simulink model "Team_46"  (R2021a)
settings: Solver=VariableStepAuto  StartTime=0.0  StopTime=1.79  RelTol=1e-3
undefined symbols (not defined in the file): D1, Delta
libraries: spsLoadFlowBusLib x5, spsThreePhaseVIMeasurementLib x4, spsThreePhaseSeriesRLCBranchLib x3, spsThreePhaseParallelRLCLoadLib x3, spsMultimeterLib x3, spsThreePhaseSourceLib x2, spsThreePhaseFaultLib x2, spsSynchronousMachinepuStandardLib x2, spsThreePhaseTransformerTwoWindingsLib x2, spsThreePhaseMutualInductanceZ1Z0Lib x2, spsThreePhaseSeriesRLCLoadLib x1, spsParallelRLCBranchLib x1
settings Model: Creator=Tanvi Purwar  LastModifiedBy=Tanvi Purwar

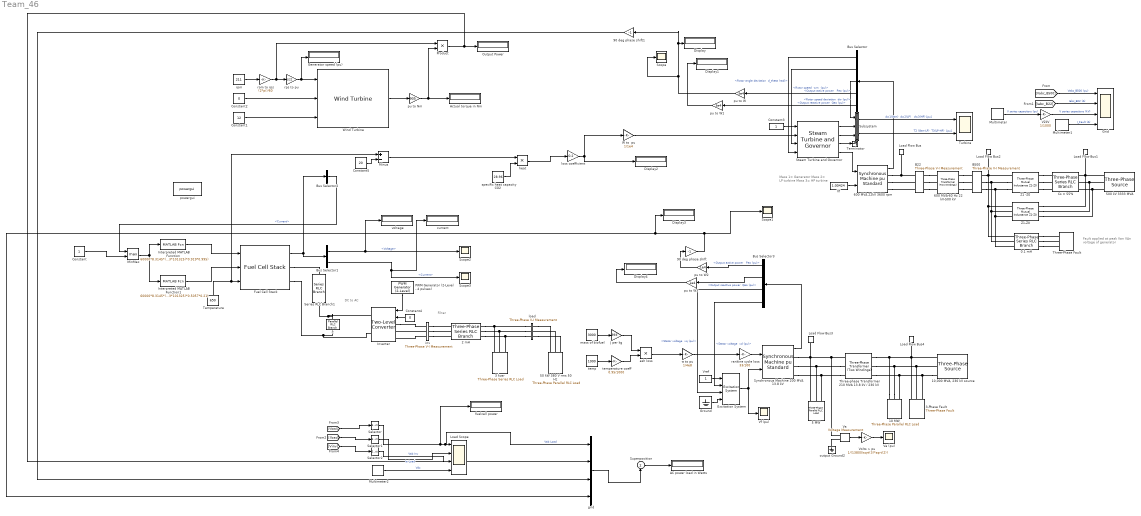
== system Team_46 ==
  note: DC to AC
  note: Mass 1= Generator
      | Mass 2= LP turbine
      | Mass 3= HP turbine
  note: Fault applied at peak Van
      | VAn voltage of generator
  note: Filter
  " mass of biofuel" : Constant  Value=3000
  0.1 mH : spsThreePhaseSeriesRLCBranchLib/Three-Phase Series RLC Branch  LConnTagsString=A|B|C  RConnTagsString=A|B|C  BranchType=L  Resistance=1.0  Inductance=0.1e-3  Capacitance=1e-6  Measurements=None
  10 MW : spsThreePhaseParallelRLCLoadLib/Three-Phase Parallel RLC Load  LConnTagsString=A|B|C  Configuration=Y (grounded)  NominalVoltage=230e3  Vabc=[1e3 1e3 1e3]  Vabcp=[1e3 1e3 1e3]  NominalFrequency=60  UnbalancedPower=off  ActivePower=10000000  InductivePower=0  CapacitivePower=0  Pabc=[10e3 9e3 11e3]  QLabc=[100 90 110]  QCabc=[100 90 110]  Pabcp=[10e3 9e3 11e3]  QLabcp=[100 90 110]  QCabcp=[100 90 110]  Measurements=None  LoadType=constant Z
  "10,000 MVA, 230 kV source" : spsThreePhaseSourceLib/Three-Phase Source  InternalConnection=Yg  VoltagePhases=off  Voltage=(230000)*1.00006  PhaseAngle=-0.77547  Voltage_phases=[25e3 25e3 25e3]/sqrt(3)  PhaseAngles_phases=[0 -120 +120]  Frequency=60  NonIdealSource=on  SpecifyImpedance=on  Resistance=0.529  Inductance=0.0140  ShortCircuitLevel=10000e6  BaseVoltage=230e3  XRratio=10  BusType=swing  Pref=0  Qref=0  Prefabc=[10e3, 10e3, 10e3]  Qrefabc=[0, 0, 0]  Qmin=-Inf  Qmax=Inf
  "2 mH " : spsThreePhaseSeriesRLCBranchLib/Three-Phase Series RLC Branch  LConnTagsString=A|B|C  RConnTagsString=A|B|C  BranchType=L  Resistance=0  Inductance=2e-3  Capacitance=inf  Measurements=None
  3 kvar : spsThreePhaseSeriesRLCLoadLib/Three-Phase Series RLC Load  LConnTagsString=A|B|C  Configuration=Delta  NominalVoltage=380  Vabc=[1e3 1e3 1e3]  Vabcp=[1e3 1e3 1e3]  NominalFrequency=50  UnbalancedPower=off  ActivePower=0  InductivePower=0  CapacitivePower=3e3  Pabc=[10e3 9e3 11e3]  QLabc=[100 90 110]  QCabc=[100 90 110]  Pabcp=[10e3 9e3 11e3]  QLabcp=[100 90 110]  QCabcp=[100 90 110]  Measurements=None  LoadType=constant Z
  3-Phase Fault : spsThreePhaseFaultLib/Three-Phase Fault  InitialStates=0  FaultA=on  FaultB=on  FaultC=on  GroundFault=on  SwitchTimes=[ 0.1 0.2]  External=off  SwitchStatus=NaN  FaultResistance=1e-3  GroundResistance=1e-3  SnubberResistance=inf  SnubberCapacitance=inf  Measurements=None
  5 MW : spsThreePhaseParallelRLCLoadLib/Three-Phase Parallel RLC Load  LConnTagsString=A|B|C  Configuration=Y (grounded)  NominalVoltage=13.8e3  Vabc=[1e3 1e3 1e3]  Vabcp=[1e3 1e3 1e3]  NominalFrequency=60  UnbalancedPower=off  ActivePower=5000000  InductivePower=0  CapacitivePower=0  Pabc=[10e3 9e3 11e3]  QLabc=[100 90 110]  QCabc=[100 90 110]  Pabcp=[10e3 9e3 11e3]  QLabcp=[100 90 110]  QCabcp=[100 90 110]  Measurements=None  LoadType=constant Z
  50 kW 380 V rms 50 Hz : spsThreePhaseParallelRLCLoadLib/Three-Phase Parallel RLC Load  LConnTagsString=A|B|C  Configuration=Delta  NominalVoltage=380  Vabc=[1e3 1e3 1e3]  Vabcp=[1e3 1e3 1e3]  NominalFrequency=50  UnbalancedPower=off  ActivePower=50e3  InductivePower=0  CapacitivePower=0  Pabc=[10e3 9e3 11e3]  QLabc=[100 90 110]  QCabc=[100 90 110]  Pabcp=[10e3 9e3 11e3]  QLabcp=[100 90 110]  QCabcp=[100 90 110]  Measurements=None  LoadType=constant Z
  500 kV 3333 MVA : spsThreePhaseSourceLib/Three-Phase Source  InternalConnection=Yg  VoltagePhases=off  Voltage=(500000)*0.99995  PhaseAngle=0.063884  Voltage_phases=[25e3 25e3 25e3]/sqrt(3)  PhaseAngles_phases=[0 -120 +120]  Frequency=60  NonIdealSource=on  SpecifyImpedance=on  Resistance=3.5  Inductance=0.1989  ShortCircuitLevel=3333e6  BaseVoltage=500e3  XRratio=21.43  BusType=swing  Pref=0  Qref=0  Prefabc=[10e3, 10e3, 10e3]  Qrefabc=[0, 0, 0]  Qmin=-Inf  Qmax=Inf
  600 MVA 22kV 3600 rpm : spsSynchronousMachinepuStandardLib/Synchronous Machine pu Standard  PresetModel=No  MechanicalLoad=Mechanical power Pm  ShowDetailedParameters=on  RotorType=Round  Units=per unit standard parameters  MeasurementBus=off  NominalParameters="[ 600e6  22e3   60 ]"  Reactances1=[ 1.65, 0.25, 0.2, 1.59, 0.46, 0.2, 0.14 ]  Reactances2="[ 1.305, 0.296, 0.252, 0.474,  0.243,  0.18 ]"  dAxisTimeConstants=Open-circuit  qAxisTimeConstants=Open-circuit  TimeConstants1="[ 4.4849  0.0681  0.1  ]"  TimeConstants2="[ 4.5, 0.04,  0.67, 0.09 ]"  TimeConstants3="[  4.49  0.0681  0.0513  ]"  TimeConstants4=[ 8.0, 0.03, 0.3371, 0.0295 ]  TimeConstants5=[ 1.01, 0.053, 0.1 ]  TimeConstants6=[ 1.3201, 0.023, 1.0, 0.07 ]  TimeConstants7="[  1.01  0.053  0.051266  ]"  TimeConstants8=[ 1.3201, 0.0231, 0.3371, 0.0295 ]  StatorResistance=0.0045  Mechanical="[ 0.8788  0 1 ]"  PolePairs=1  InitialConditions=[0 -120.067 0.00256993 0.00256993 0.00256993 -120.066 -240.066 -0.0663631 1.00424]  SetSaturation=off  Saturation=[0.6404,0.7127,0.8441,0.9214,0.9956,1.082,1.19,1.316,1.457;0.7,0.7698,0.8872,0.9466,0.9969,1.046,1.1,1.151,1.201]  LoadFlowParameters=[1 0 0 0 0]  TsPowergui=0  TsBlock=-1  IterativeModel=Trapezoidal non iterative  IterativeDiscreteModel=Trapezoidal non iterative  BusType=PV  Pref=0  Qref=0  Qmin=-Inf  Qmax=Inf  PLF=0  QLF=0
      settings: SourceProductBaseCode=PS
  600 MVA-60 Hz 22 kV-500 kV : spsThreePhaseTransformerTwoWindingsLib/Three-Phase Transformer (Two Windings)  Winding1Connection=Delta (D1)  Winding2Connection=Yg  CoreType=Three single-phase transformers  SetSaturation=off  Hysteresis=off  DataFile='hysteresis'  SetInitialFlux=off  Measurements=None  UNITS=pu  NominalPower="[ 600e6   60 ]"  Winding1="[ 22e3  0.06/100 0 ]"  Winding2="[ 500e3  0.06/100  0.12]"  Rm=500  Lm=500  L0=0.5  Saturation="[ 0,0  ;  0.005,1.2  ;  1.0,1.4 ]"  InitialFluxes=[ 0.8 , -0.8 , 0.7 ]  BreakLoop=off  DiscreteSolver=Trapezoidal iterative  DataType=off  TransfoNumber=0
  90 deg phase shift : Gain  Gain=-1
  90 deg phase shift1 : Gain  Gain=-1
  AC power load in Watts : Display
  Actual torque in Nm : Display
  B22 : spsThreePhaseVIMeasurementLib/Three-Phase V-I Measurement  VoltageMeasurement=no  SetLabelV=on  LabelV=Vabc_B22  Vpu=off  VpuLL=off  CurrentMeasurement=yes  SetLabelI=on  LabelI=Iabc_B22  Ipu=off  Pbase=100e6  Vbase=500e3  OutputType=Complex  PhasorSimulation=off  PSBequivalent=0
  B500 : spsThreePhaseVIMeasurementLib/Three-Phase V-I Measurement  VoltageMeasurement=phase-to-ground  SetLabelV=on  LabelV=Vabc_B500  Vpu=on  VpuLL=off  CurrentMeasurement=no  SetLabelI=on  LabelI=Iabc_B500  Ipu=on  Pbase=100e6  Vbase=500e3  OutputType=Complex  PhasorSimulation=off  PSBequivalent=0
  Bus Selector : BusSelector  OutputSignals="Mechanical.Rotor angle deviation  d_theta (rad),Mechanical.Rotor speed  wm  (pu),Mechanical.Rotor speed deviation  dw (pu),Output active power   Peo (pu),Output reactive power  Qeo (pu)"
  Bus Selector1 : BusSelector  OutputSignals=Voltage,Current
  Bus Selector2 : BusSelector  OutputSignals=Current
  Bus Selector3 : BusSelector  OutputSignals="Output active power   Peo (pu),Output reactive power  Qeo (pu),dq0 components.Stator voltage  vq (pu),dq0 components.Stator voltage  vd (pu)"
  C : spsParallelRLCBranchLib/Parallel RLC Branch  LConnTagsString=a  RConnTagsString=__new0  BranchType=C  Resistance=inf  Inductance=inf  SetiL0=off  InitialCurrent=0  Capacitance=5000e-06  Setx0=on  InitialVoltage=775  Measurements=Branch voltage
  Constant : Constant
  Constant1 : Constant  Value=12
  Constant2 : Constant  Value=0
  Constant3 : Constant
  Constant4 : Constant  Value=0
  Constant5 : Constant  Value=20
  Cs = 55% : spsThreePhaseSeriesRLCBranchLib/Three-Phase Series RLC Branch  LConnTagsString=A|B|C  RConnTagsString=A|B|C  BranchType=C  Resistance=[]  Inductance=[]  Capacitance=1/(0.55*0.080*(500e3^2/100e6))/(2*pi*60)  Measurements=Branch voltages
  Display{,1..4} (5 alike) : Display
  Excitation System : spsExcitationSystemLib/Excitation System  tr=20e-3  reg=[ 300, 0.001 ]  exc=[ 1, 0 ]  tgr=[ 0, 0 ]  damp=[ 0.001, 0.1 ]  sat=[ 0, 0 ]  lim=[ -11.5, 11.5, 0 ]  v0=[1,1.29071]
      settings: SourceProductBaseCode=PS
  Fuel Cell Stack : spsFuelCellStackLib/Fuel Cell Stack  PresetModel=PEMFC - 6 kW - 45 Vdc  FcType=0  Detailed=Detailed  Eoc=[65,63]  NomVI=[133.3,45]  EndVI=[225,37]  Nc=65  n=55  TOp=65  AirFr=300  SuppPress=[1.5,1]  Comp=[99.95,21,1]  SignX=off  SignY=off  FlowRateH2=on  FlowRateAir=on  SystemTemp=on  SystemPH2=off  SystemPAir=off  FCDyn=off  FC_tau=1  Peak_O2=80  V_Under=10
      settings: SourceProductBaseCode=PS
  Generator speed (pu) : Display
  Grid : Scope  NumInputPorts=4
  Ground : Ground
  Interpreted MATLAB Function : MATLABFcn  MATLABFcn=60000*8.3145*(273+95)*400*u(1)/(2*96485*(3*101325)*0.919*0.995)
  Interpreted MATLAB Function1 : MATLABFcn  MATLABFcn=60000*8.3145*(273+95)*400*u(1)/(4*96485*(3*101325)*0.5057*0.21)
  Inverter : spsTwoLevelConverterLib/Two-Level Converter  ModelType=Switching devices  Ron=1e-3  Rs=1e6  Cs=inf  Vforward=[0,0]  Ron_Diode=1e-3  Rs_Diode=1e6  Cs_Diode=inf  Vf_Diode=1e-3  Rs_CurrentSource=inf
      settings: SourceProductBaseCode=PS
  J per kg : Gain  Gain=393
  Load Scope : Scope  NumInputPorts=4
  Load Flow Bus : spsLoadFlowBusLib/Load Flow Bus  LConnTagsString=a  Phases=single  Connectors=on one side  ID=B22  Vbase=22e3  Vref=1  Vangle=0  VLF=1  VLFb=1  VLFc=1  angleLF=-30.07  angleLFb=0  angleLFc=0
      settings: AttributesFormatString=%<ID>\n%<Vbase>V\n%<VLF>pu\n%<angleLF>deg.  SourceProductBaseCode=PS
  Load Flow Bus1 : spsLoadFlowBusLib/Load Flow Bus  LConnTagsString=a  Phases=single  Connectors=on one side  ID=BSRC  Vbase=500e3  Vref=1  Vangle=0  VLF=1  VLFb=1  VLFc=1  angleLF=0  angleLFb=0  angleLFc=0
      settings: AttributesFormatString=%<ID>\n%<Vbase>V\n%<VLF>pu\n%<angleLF>deg.  SourceProductBaseCode=PS
  Load Flow Bus2 : spsLoadFlowBusLib/Load Flow Bus  LConnTagsString=a  Phases=single  Connectors=on one side  ID=B500  Vbase=500e3  Vref=1  Vangle=0  VLF=0.9999  VLFb=1  VLFc=1  angleLF=-0.05226  angleLFb=0  angleLFc=0
      settings: AttributesFormatString=%<ID>\n%<Vbase>V\n%<VLF>pu\n%<angleLF>deg.  SourceProductBaseCode=PS
  Load Flow Bus3 : spsLoadFlowBusLib/Load Flow Bus  LConnTagsString=a  Phases=single  Connectors=on one side  ID=B1  Vbase=13.8e3  Vref=1  Vangle=0  VLF=1  VLFb=1  VLFc=1  angleLF=-23.67  angleLFb=0  angleLFc=0
      settings: AttributesFormatString=%<ID>\n%<Vbase>V\n%<VLF>pu\n%<angleLF>deg.  SourceProductBaseCode=PS
  Load Flow Bus4 : spsLoadFlowBusLib/Load Flow Bus  LConnTagsString=a  Phases=single  Connectors=on one side  ID=B2  Vbase=230e3  Vref=1  Vangle=0  VLF=1  VLFb=1  VLFc=1  angleLF=0  angleLFb=0  angleLFc=0
      settings: AttributesFormatString=%<ID>\n%<Vbase>V\n%<VLF>pu\n%<angleLF>deg.  SourceProductBaseCode=PS
  MinMax : MinMax  Function=max  Inputs=2
  Minus : Sum  Inputs=+-
  Multimeter : spsMultimeterLib/Multimeter  PhasorSimulation=off  OutputType=Complex  sel=[1 2 3]  L=7  Gain=[1 1 1]  yselected={'Ub1: Cs = 55%','Ub2: Cs = 55%','Ub3: Cs = 55%'};  PSBOutputType=1  PSBequivalent=0  AxesSetting=[0,0.1,-100,100]  Display=0  SavedBlockNames=-11
  Multimeter1 : spsMultimeterLib/Multimeter  PhasorSimulation=off  OutputType=Complex  sel=[5 6 7]  L=7  Gain=[1 1 1]  yselected={'Ib: Three-Phase Fault/Fault A','Ib: Three-Phase Fault/Fault B','Ib: Three-Phase Fault/Fault C'};  PSBOutputType=1  PSBequivalent=0  AxesSetting=[0,0.1,-100,100]  Display=0  SavedBlockNames=-11
  Multimeter2 : spsMultimeterLib/Multimeter  PhasorSimulation=off  OutputType=Complex  sel=1  L=7  Gain=0  yselected={}  PSBOutputType=1  PSBequivalent=0  AxesSetting=[0,0.1,-100,100]  Display=0  SavedBlockNames=-11
  Output Power : Display
  PWM Generator (2-Level - 4 pulses) : spsPWMGenerator2LevelLib/PWM Generator (2-Level)  ModulatorType=Three-phase bridge (6 pulses)  ModulatorMode=Unsynchronized  Fc=2000  Pc=90  nF=27  MinMax="[ -1  1 ]"  SamplingTechnique=Natural  ModulatingSignals=on  m=0.8  Freq=50  Phase=0  Ts=4e-6  ShowCarrierOutport=off
  Product : Product
  Scope{,1..3} (4 alike) : Scope
  Selector : Selector  IndexMode=Zero-based  InputPortWidth=3  IndexOptions=Index vector (dialog)  Indices=0  OutputSizes=1
  Selector1 : Selector  IndexMode=Zero-based  InputPortWidth=3  IndexOptions=Index vector (dialog)  Indices=1  OutputSizes=1
  Selector2 : Selector  IndexMode=Zero-based  InputPortWidth=3  IndexOptions=Index vector (dialog)  Indices=2  OutputSizes=1
  Series RLC Branch1 : spsSeriesRLCBranchLib/Series RLC Branch  LConnTagsString=__new0  RConnTagsString=__new0  BranchType=R  Resistance=1  Inductance=1e-3  SetiL0=off  InitialCurrent=0  Capacitance=1e-6  Setx0=off  InitialVoltage=0  Measurements=None
  Steam Turbine and Governor : spsSteamTurbineandGovernorLib/Steam Turbine and Governor  gentype=Tandem-compound (multi-mass)  reg1="[ 1  0.05    0 ]"  reg2="[ 0.001  0.15 ]"  reg3="[ -0.1  0.1  0  4.496]"  N=3600  turb1="[ 0  10   3.3   0.5   ]"  turb2="[ 0.5   0.5   0  0 ]"  HA="[  1.5498   0.24894  0  0 ]"  KA="[  83.47  42.702  0  0 ]"  DA="[  0.3104  0.05  0  0 ]*8"  ini1=250.35/555  ini2=[1.88924e-008,-120.067]
      settings: SourceProductBaseCode=PS
  Subsystem : Subsystem
  Superposition : Sum  Inputs=|+
  Synchronous Machine 200 MVA 13.8 kV : spsSynchronousMachinepuStandardLib/Synchronous Machine pu Standard  PresetModel=No  MechanicalLoad=Mechanical power Pm  ShowDetailedParameters=on  RotorType=Salient-pole  Units=per unit standard parameters  MeasurementBus=off  NominalParameters="[ 200E6  13800   60 ]"  Reactances1=[ 31 32 33 34 35 36 37 ]  Reactances2=[ 1.305, 0.296, 0.252, 0.474, 0.243, 0.18 ]  dAxisTimeConstants=Short-circuit  qAxisTimeConstants=Open-circuit  TimeConstants1=[]  TimeConstants2=[]  TimeConstants3=[]  TimeConstants4=[]  TimeConstants5=[ 1.01, 0.053, 0.1 ]  TimeConstants6=[]  TimeConstants7=[]  TimeConstants8=[]  StatorResistance=2.8544e-3  Mechanical=[ 3.2 0 2]  PolePairs=2  InitialConditions=[0 -94.2826 0.750185 0.750185 0.750185 -24.943 -144.943 95.057 1.29071]  SetSaturation=off  Saturation=[0.6404,0.7127,0.8441,0.9214,0.9956,1.082,1.19,1.316,1.457;0.7,0.7698,0.8872,0.9466,0.9969,1.046,1.1,1.151,1.201]  LoadFlowParameters=[1 150000000 0 0]  TsPowergui=0  TsBlock=-1  IterativeModel=Trapezoidal non iterative  IterativeDiscreteModel=Trapezoidal non iterative  BusType=PV  Pref=150000000  Qref=0  Qmin=-Inf  Qmax=Inf  PLF=0  QLF=0
      settings: SourceProductBaseCode=PS
  Temperature : Constant  Value=650
  Terminator : Terminator
  Three-Phase Fault : spsThreePhaseFaultLib/Three-Phase Fault  InitialStates=0  FaultA=on  FaultB=on  FaultC=on  GroundFault=on  SwitchTimes="[ (1+1/3 )/60   (1+1/3)/60+0.0169 ]"  External=off  SwitchStatus=NaN  FaultResistance=0.001  GroundResistance=0.001  SnubberResistance=1e5  SnubberCapacitance=inf  Measurements=Fault currents
  Three-phase Transformer 210 MVA 13.8 kV / 230 kV : spsThreePhaseTransformerTwoWindingsLib/Three-Phase Transformer (Two Windings)  Winding1Connection=Delta (D1)  Winding2Connection=Yg  CoreType=Three single-phase transformers  SetSaturation=off  Hysteresis=off  DataFile='hysteresis'  SetInitialFlux=off  Measurements=None  UNITS=pu  NominalPower=[ 210e6 60 ]  Winding1="[ 13.8e3 0.0027  0.08]"  Winding2=[ 230e3 0.0027 0.08]  Rm=500  Lm=500  L0=0.5  Saturation="[ 0,0  ;  0.005,1.2  ;  1.0,1.4 ]"  InitialFluxes=[ 0.8 , -0.8 , 0.7 ]  BreakLoop=off  DiscreteSolver=Trapezoidal iterative  DataType=off  TransfoNumber=0
  Turbine : Scope  NumInputPorts=2
  V2kV : Gain  Gain=1/1000
  Va : spsVoltageMeasurementLib/Voltage Measurement  Tag=PoWeRsYsTeMmEaSuReMeNt  PhasorSimulation=off  OutputType=Magnitude  PSBequivalent=0
  Va (pu) : Scope
  Vf : Constant  Value=1.00424
  Vf (pu) : Scope
  Volts > pu : Gain  Gain=1/(13800/sqrt(3)*sqrt(2))  SaturateOnIntegerOverflow=on  OutDataTypeStr=Inherit: Same as input  ParamDataTypeStr=Inherit: Same as input
  Vref : Constant
  W to  pu : Gain  Gain=1/1e4
  Wind Turbine : spsWindTurbineLib/Wind Turbine  Pnom=20e3  Pelec_base=20e3/0.9  wind_base=12  P_wind_base=1  speed_nom=1  pitch_angle=0  c1_c6="[0.51763          116          0.4            5           21     0.006795]"  cp_nom=0.48  lambda_nom=8.1
      settings: SourceProductBaseCode=PS
  Z1 -Z0 : spsThreePhaseMutualInductanceZ1Z0Lib/Three-Phase Mutual Inductance Z1-Z0  LConnTagsString=a|b|c  RConnTagsString=A|B|C  PositiveSequence="[ 0.0074   0.080/(2*pi*60) ]*(500e3^2/100e6)"  ZeroSequence="[ 0.022   0.240/(2*pi*60) ]*(500e3^2/100e6)"
      settings: AttributesFormatString=\n  SourceProductBaseCode=PS
  "Z1-Z0 " : spsThreePhaseMutualInductanceZ1Z0Lib/Three-Phase Mutual Inductance Z1-Z0  LConnTagsString=a|b|c  RConnTagsString=A|B|C  PositiveSequence="[ 0.0067   0.0739/(2*pi*60) ]*(500e3^2/100e6)"  ZeroSequence="[ 0.0186   0.210/(2*pi*60) ]*(500e3^2/100e6)"
      settings: AttributesFormatString=\n  SourceProductBaseCode=PS
  ash loss : Product
  current : Display
  fuelcell power : Display
  grid : BusCreator  Inputs=4
  heat : Product
  inv : spsThreePhaseVIMeasurementLib/Three-Phase V-I Measurement  VoltageMeasurement=phase-to-phase  SetLabelV=on  LabelV=Vinv  Vpu=off  VpuLL=off  CurrentMeasurement=no  SetLabelI=on  LabelI=Iload  Ipu=off  Pbase=1e3  Vbase=380  OutputType=Magnitude  PhasorSimulation=off  PSBequivalent=0
  load : spsThreePhaseVIMeasurementLib/Three-Phase V-I Measurement  VoltageMeasurement=phase-to-phase  SetLabelV=on  LabelV=Vload  Vpu=off  VpuLL=off  CurrentMeasurement=yes  SetLabelI=on  LabelI=Iload  Ipu=off  Pbase=1e3  Vbase=380  OutputType=Magnitude  PhasorSimulation=off  PSBequivalent=0
  loss coefficient : Gain  Gain=0.2
  output Ground2 : spsGroundLib/Ground  LConnTagsString=a
  powergui : spspowerguiLib/powergui  Priority=1  SimulationMode=Discrete  SampleTime=4e-6  frequency=60  Iterations=50  frequencyindice=60  Pbase=100e6  ErrMax=1e-4  UnitsV=kV  UnitsW=MW  buscounter=0  FunctionMessages=off  echomessages=off  EnableUseOfTLC=off  CurrentSourceSwitches=off  DisableSnubberDevices=off  DisableRonSwitches=off  DisableVfSwitches=off  DisplayEquations=off  AutomaticDiscreteSolvers=off  SolverType=Tustin/Backward Euler (TBE)  Interpol=off  ExternalGateDelay=off  methode=off  Ts=100  x0status=blocks  SPID=off  SwTol=0  HookPort=off  NonlinearTolerance=1e-4  nMaxIteration=100  ContinueOnMaxIteration=off  RestoreLinks=warning  ResistiveCurrentMeasurement=off  Frange=[0:2:500]  Ylog=off  Xlog=on  ShowGrid=off  save=off  variable=ZData  structure=0  ZoomFFT=off  StartTime=0.0  cycles=1  DisplayStyle=1  fundamental=60  FreqAxis=off  MaxFrequency=1000  frequencyindicesteady=1  RmsSteady=1  display=off
  pu to Nm : Gain  Gain=905
  pu to W : Gain  Gain=3e4
  pu to W1 : Gain  Gain=3e4
  pu to W2 : Gain  Gain=1e4
  pu to W3 : Gain  Gain=1e4
  rankine cycle loss : Gain  Gain=33/100
  rpm : Constant  Value=211
  rpm to rps : Gain  Gain=(2*pi)/60
  rps to pu : Gain  Gain=1/22
  specific heat capacity CO2 : Constant  Value=28.96
  temp : Constant  Value=1000
  temperature coeff : Gain  Gain=0.95/1000
  voltage : Display
  w to pu : Gain  Gain=1/4e8
  wires:
  Constant2/1 -> Wind Turbine/2
  Constant1/1 -> Wind Turbine/3
  rpm/1 -> rpm to rps/1
  rpm to rps/1 -> Product/1, rps to pu/1
  rps to pu/1 -> Generator speed (pu)/1, Wind Turbine/1
  Wind Turbine/1 -> pu to Nm/1
  pu to Nm/1 -> Product/2, Actual torque in Nm/1
  Product/1 -> Output Power/1, grid/2
  MinMax/1 -> Interpreted MATLAB Function1/1, Interpreted MATLAB Function/1
  Bus Selector1/2 -> Scope3/1, current/1  "<Current>"
  Interpreted MATLAB Function1/1 -> Fuel Cell Stack/2
  Constant/1 -> MinMax/2
  Bus Selector2/1 -> MinMax/1  "<Current>"
  Bus Selector1/1 -> Scope2/1, voltage/1  "<Voltage>"
  Interpreted MATLAB Function/1 -> Fuel Cell Stack/1
  Fuel Cell Stack/1 -> Bus Selector1/1, Bus Selector2/1
  Temperature/1 -> Fuel Cell Stack/3, Minus/1
  Bus Selector/5 -> pu to W1/1  "<Output reactive power  Qeo (pu)>"
  pu to W1/1 -> Display1/1
  Steam Turbine and Governor/3 -> Terminator/1
  Multimeter/1 -> V2kV/1  "V series capacitors (pu)"
  Steam Turbine and Governor/2 -> Subsystem/3(In3)
  [Iabc_B22] -> Grid/2  "Iabc_B22 (A)"
  [Vabc_B500] -> Grid/1  "Vabc_B500 (pu)"
  V2kV/1 -> Grid/3  "V series capacitors (kV)"
  Bus Selector/3 -> Subsystem/1(In1)  "<Rotor speed deviation  dw (pu)>"
  Bus Selector/4 -> pu to W/1  "<Output active power   Peo (pu)>"
  Steam Turbine and Governor/4 -> 600 MVA 22kV 3600 rpm/1
  Vf/1 -> 600 MVA 22kV 3600 rpm/2
  pu to W/1 -> 90 deg phase shift1/1, Display/1, Scope/1
  Steam Turbine and Governor/1 -> Subsystem/2(In2)
  Subsystem/1(dw_123) -> Turbine/1  "dw1(Gen)  dw2(LP)   dw3(HP) [pu]"
  Bus Selector/2 -> Steam Turbine and Governor/3  "<Rotor speed  wm  (pu)>"
  600 MVA 22kV 3600 rpm/1 -> Bus Selector/1
  Multimeter1/1 -> Grid/4  "I_Fault (A)"
  Bus Selector/1 -> Steam Turbine and Governor/4  "<Rotor angle deviation  d_theta (rad)>"
  Subsystem/2(T_23) -> Turbine/2  "T2 (Gen-LP)  T3(LP-HP)  [pu]"
  Constant3/1 -> Steam Turbine and Governor/1
  loss coefficient/1 -> W to  pu/1, Display2/1
  W to  pu/1 -> Steam Turbine and Governor/2
  J per kg/1 -> ash loss/1
  " mass of biofuel"/1 -> J per kg/1
  Bus Selector3/2 -> pu to W3/1  "<Output reactive power  Qeo (pu)>"
  w to pu/1 -> rankine cycle loss/1
  temperature coeff/1 -> ash loss/2
  Bus Selector3/3 -> Excitation System/3  "<Stator voltage  vq (pu)>"
  Va/1 -> Volts > pu/1
  Bus Selector3/1 -> pu to W2/1  "<Output active power   Peo (pu)>"
  ash loss/1 -> w to pu/1
  rankine cycle loss/1 -> Synchronous Machine 200 MVA 13.8 kV/1
  Bus Selector3/4 -> Excitation System/2  "<Stator voltage  vd (pu)>"
  Excitation System/1 -> Vf (pu)/1, Synchronous Machine 200 MVA 13.8 kV/2
  Synchronous Machine 200 MVA 13.8 kV/1 -> Bus Selector3/1
  temp/1 -> temperature coeff/1
  Ground/1 -> Excitation System/4
  pu to W3/1 -> Display4/1
  Volts > pu/1 -> Va (pu)/1
  Vref/1 -> Excitation System/1
  Selector2/1 -> Load Scope/3  "Vab Inv"
  PWM Generator (2-Level - 4 pulses)/1 -> Inverter/1
  Multimeter2/1 -> Load Scope/4  "Vdc"
  [Vload] -> Selector/1
  Selector/1 -> fuelcell power/1, grid/1, Load Scope/1  "Vab Load"
  Selector1/1 -> Load Scope/2  "Ia Load"
  Constant4/1 -> Inverter/2
  [Vinv] -> Selector2/1
  [Iload] -> Selector1/1
  grid/1 -> Superposition/1
  Superposition/1 -> AC power load in Watts/1
  90 deg phase shift/1 -> grid/4, Display3/1, Scope1/1
  pu to W2/1 -> 90 deg phase shift/1
  Constant5/1 -> Minus/2
  Minus/1 -> heat/1
  specific heat capacity CO2/1 -> heat/2
  heat/1 -> loss coefficient/1
  90 deg phase shift1/1 -> grid/3
  connections:
  Fuel Cell Stack/RConn1 -- Series RLC Branch1/LConn1
  Z1 -Z0/LConn3 -- "Z1-Z0 "/LConn3 -- 0.1 mH/LConn3 -- B500/RConn3
  Load Flow Bus/LConn1 -- 600 MVA 22kV 3600 rpm/RConn1 -- B22/LConn1
  Load Flow Bus1/LConn1 -- "Z1-Z0 "/RConn1 -- 500 kV 3333 MVA/RConn1 -- Cs = 55%/LConn1
  B500/RConn1 -- Load Flow Bus2/LConn1 -- Z1 -Z0/LConn1 -- 0.1 mH/LConn1 -- "Z1-Z0 "/LConn1
  Z1 -Z0/LConn2 -- "Z1-Z0 "/LConn2 -- 0.1 mH/LConn2 -- B500/RConn2
  Cs = 55%/LConn3 -- "Z1-Z0 "/RConn3 -- 500 kV 3333 MVA/RConn3
  Cs = 55%/LConn2 -- "Z1-Z0 "/RConn2 -- 500 kV 3333 MVA/RConn2
  600 MVA 22kV 3600 rpm/RConn2 -- B22/LConn2
  B22/RConn2 -- 600 MVA-60 Hz 22 kV-500 kV/LConn2
  0.1 mH/RConn2 -- Three-Phase Fault/LConn2
  0.1 mH/RConn1 -- Three-Phase Fault/LConn1
  B22/RConn3 -- 600 MVA-60 Hz 22 kV-500 kV/LConn3
  0.1 mH/RConn3 -- Three-Phase Fault/LConn3
  600 MVA 22kV 3600 rpm/RConn3 -- B22/LConn3
  600 MVA-60 Hz 22 kV-500 kV/RConn1 -- B500/LConn1
  Z1 -Z0/RConn1 -- Cs = 55%/RConn1
  B22/RConn1 -- 600 MVA-60 Hz 22 kV-500 kV/LConn1
  600 MVA-60 Hz 22 kV-500 kV/RConn3 -- B500/LConn3
  Z1 -Z0/RConn2 -- Cs = 55%/RConn2
  Z1 -Z0/RConn3 -- Cs = 55%/RConn3
  600 MVA-60 Hz 22 kV-500 kV/RConn2 -- B500/LConn2
  "10,000 MVA, 230 kV source"/RConn3 -- Three-phase Transformer 210 MVA 13.8 kV / 230 kV/RConn3 -- 10 MW/LConn3 -- 3-Phase Fault/LConn3
  Load Flow Bus3/LConn1 -- Synchronous Machine 200 MVA 13.8 kV/RConn1 -- 5 MW/LConn1 -- Three-phase Transformer 210 MVA 13.8 kV / 230 kV/LConn1 -- Va/LConn1
  Three-phase Transformer 210 MVA 13.8 kV / 230 kV/LConn3 -- Synchronous Machine 200 MVA 13.8 kV/RConn3 -- 5 MW/LConn3
  10 MW/LConn1 -- Three-phase Transformer 210 MVA 13.8 kV / 230 kV/RConn1 -- 3-Phase Fault/LConn1 -- "10,000 MVA, 230 kV source"/RConn1 -- Load Flow Bus4/LConn1
  Three-phase Transformer 210 MVA 13.8 kV / 230 kV/LConn2 -- Synchronous Machine 200 MVA 13.8 kV/RConn2 -- 5 MW/LConn2
  10 MW/LConn2 -- Three-phase Transformer 210 MVA 13.8 kV / 230 kV/RConn2 -- 3-Phase Fault/LConn2 -- "10,000 MVA, 230 kV source"/RConn2
  output Ground2/LConn1 -- Va/LConn2
  load/LConn1 -- "2 mH "/RConn1 -- 3 kvar/LConn1
  load/LConn2 -- "2 mH "/RConn2 -- 3 kvar/LConn2
  load/LConn3 -- "2 mH "/RConn3 -- 3 kvar/LConn3
  inv/LConn2 -- Inverter/LConn2
  load/RConn3 -- 50 kW 380 V rms 50 Hz/LConn3
  50 kW 380 V rms 50 Hz/LConn2 -- load/RConn2
  inv/RConn2 -- "2 mH "/LConn2
  Inverter/LConn1 -- inv/LConn1
  inv/RConn1 -- "2 mH "/LConn1
  load/RConn1 -- 50 kW 380 V rms 50 Hz/LConn1
  inv/RConn3 -- "2 mH "/LConn3
  inv/LConn3 -- Inverter/LConn3
  C/LConn1 -- Inverter/RConn1 -- Series RLC Branch1/RConn1
  Fuel Cell Stack/RConn2 -- Inverter/RConn2 -- C/RConn1

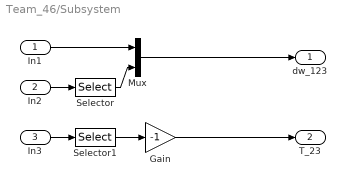
== system Team_46/Subsystem ==
  In1 : Inport
  In2 : Inport  Port=2
  In3 : Inport  Port=3
  Gain : Gain  Gain=-1  SaturateOnIntegerOverflow=on  OutDataTypeStr=Inherit: Same as input  ParamDataTypeStr=Inherit: Same as input
  Mux : Mux  Inputs=2
  Selector : Selector  InputPortWidth=4  IndexOptions=Index vector (dialog)  Indices=[4 3]  OutputSizes=1
  Selector1 : Selector  InputPortWidth=4  IndexOptions=Index vector (dialog)  Indices=[4 3]  OutputSizes=1
  dw_123 : Outport  VectorParamsAs1DForOutWhenUnconnected=off
  T_23 : Outport  Port=2  VectorParamsAs1DForOutWhenUnconnected=off
  wires:
  Selector/1 -> Mux/2
  Mux/1 -> dw_123/1
  In1/1 -> Mux/1
  In2/1 -> Selector/1
  In3/1 -> Selector1/1
  Selector1/1 -> Gain/1
  Gain/1 -> T_23/1
